simulink model "ext_mode_example"  (Simulink 7.0)
settings: Solver=FixedStepDiscrete  StartTime=0.0  StopTime=60  FixedStep=.1  RelTol=1e-3
undefined symbols (not defined in the file): A, B
settings Model: Creator=colinlea  LastModifiedBy=colinlea  SimulationMode=external
settings SolverCC: PositivePriorityOrder=on
settings DataIOCC: SaveOutput=off  SaveTime=off
settings RTWCC: ProcessScript=grt_make_rtw_hook
settings GRTTargetCC: ExtMode=on

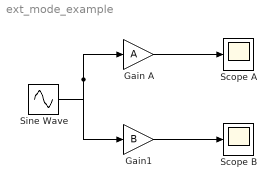
== system ext_mode_example ==
  Gain A : Gain  Gain=A  ParameterDataType=sfix(16)  ParameterScaling=2^0  OutDataType=sfix(16)  OutScaling=2^0
  Gain1 : Gain  Gain=B  ParameterDataType=sfix(16)  ParameterScaling=2^0  OutDataType=sfix(16)  OutScaling=2^0
  Scope A : Scope
      settings: YMin=-0.5  YMax=0.5
  Scope B : Scope
      settings: YMin=-3.5  YMax=3.5
  Sine Wave : Sin  SampleTime=0
  wires:
  Sine Wave/1 -> Gain A/1, Gain1/1
  Gain A/1 -> Scope A/1
  Gain1/1 -> Scope B/1
